simulink model "CS2"  (R2018b)
settings: Solver=VariableStepAuto  StartTime=0.0  StopTime=10.0  RelTol=1e-3
settings Model: Creator=bogda  LastModifiedBy=bogda

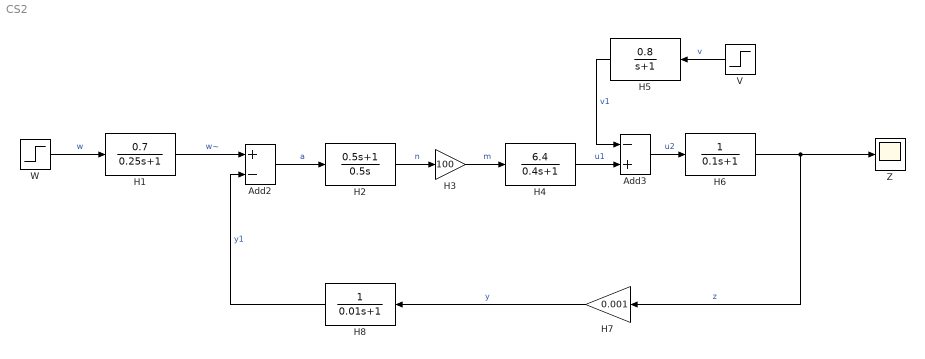
== system CS2 ==
  Add2 : Sum  Inputs=+-
  Add3 : Sum  Inputs=-+
  H1 : TransferFcn  Numerator=[0.7]  Denominator=[0.25 1]
  H2 : TransferFcn  Numerator=[0.5 1]  Denominator=[0.5 0]
  H3 : Gain  Gain=100
  H4 : TransferFcn  Numerator=[6.4]  Denominator=[0.4 1]
  H5 : TransferFcn  Numerator=[0.8]  Denominator=[1 1]
  H6 : TransferFcn  Denominator=[0.1 1]
  H7 : Gain  Gain=0.001
  H8 : TransferFcn  Denominator=[0.01 1]
  V : Step  Time=0  After=1250  SampleTime=0
  W : Step  Time=0  After=10  SampleTime=0
  Z : Scope
  wires:
  H6/1 -> H7/1, Z/1  "z"
  H5/1 -> Add3/1  "v1"
  V/1 -> H5/1  "v"
  Add3/1 -> H6/1  "u2"
  H4/1 -> Add3/2  "u1"
  H2/1 -> H3/1  "n"
  W/1 -> H1/1  "w"
  Add2/1 -> H2/1  "a"
  H8/1 -> Add2/2  "y1"
  H1/1 -> Add2/1  "w~"
  H3/1 -> H4/1  "m"
  H7/1 -> H8/1  "y"
